simulink model "ACCmpr_VD"  (R2016b)
settings: configuration reference "CodeGenConfigSet" (kept outside this file)
values from neighbouring files (symbols this model uses):
  AC_trqMaxAC_C = Calibration.Parameter    [init_ACCmpr_VD.m]
  AirC_trqCmprMax_C = Calibration.Parameter    [init_ACCmpr_VD.m]
  AirC_trqCmprMin_C = Calibration.Parameter    [init_ACCmpr_VD.m]
settings Model: Creator=胡炎林  LastModifiedBy=lenovo
settings ConfigSetRef: SourceLocation=Base Workspace

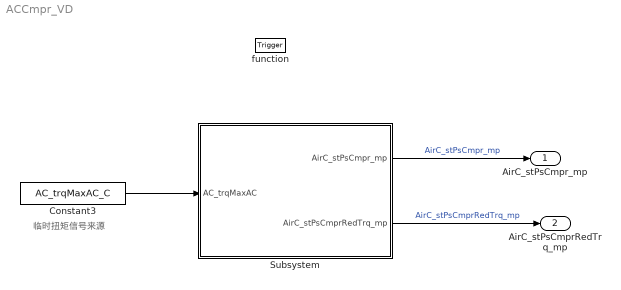
== system ACCmpr_VD ==
  note: 临时扭矩信号来源
  function : TriggerPort  TriggerType=function-call  VariantControl=Variant
  Constant3 : Constant  Value=AC_trqMaxAC_C
  Subsystem : Subsystem
  AirC_stPsCmpr_mp : Outport  Description=Measuring point for the digital output to the ACompressor actuator before error handling  OutMin=0  OutMax=1  OutDataTypeStr=boolean
  AirC_stPsCmprRedTrq_mp : Outport  Description=Measuring point for the Reduce torque instruction to the AC compressor before error handling  Port=2  OutMin=0  OutMax=1  OutDataTypeStr=boolean
  wires:
  Constant3/1 -> Subsystem/1(AC_trqMaxAC)
  Subsystem/1(AirC_stPsCmpr_mp) -> AirC_stPsCmpr_mp/1  "AirC_stPsCmpr_mp"
  Subsystem/2(AirC_stPsCmprRedTrq_mp) -> AirC_stPsCmprRedTrq_mp/1  "AirC_stPsCmprRedTrq_mp"

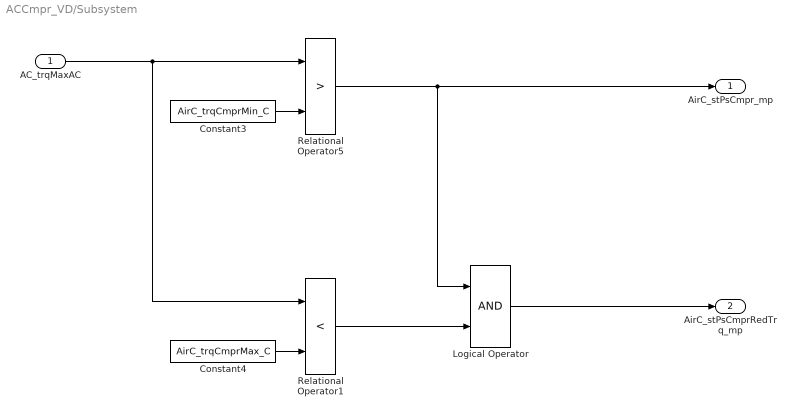
== system ACCmpr_VD/Subsystem ==
  AC_trqMaxAC : Inport
  Constant3 : Constant  Value=AirC_trqCmprMin_C
  Constant4 : Constant  Value=AirC_trqCmprMax_C
  Logical Operator : Logic  OutDataTypeStr=boolean
  Relational Operator1 : RelationalOperator  Operator=<  OutDataTypeStr=boolean  RndMeth=Simplest  InputSameDT=on
  Relational Operator5 : RelationalOperator  Operator=>  OutDataTypeStr=boolean  RndMeth=Simplest  InputSameDT=on
  AirC_stPsCmpr_mp : Outport
  AirC_stPsCmprRedTrq_mp : Outport  Port=2
  wires:
  Constant3/1 -> Relational Operator5/2
  Relational Operator1/1 -> Logical Operator/2
  Relational Operator5/1 -> AirC_stPsCmpr_mp/1, Logical Operator/1
  Logical Operator/1 -> AirC_stPsCmprRedTrq_mp/1
  Constant4/1 -> Relational Operator1/2
  AC_trqMaxAC/1 -> Relational Operator1/1, Relational Operator5/1
